simulink model "Linear_acceleration_70"  (R2022a)
settings: Solver=VariableStepAuto  StartTime=0.0  StopTime=inf  RelTol=1e-3
model workspace (MAT data in the model file):
  ratio0 = 2
  ua0 = 4.608
  ua_max = 70
undefined symbols (not defined in the file): CA, f, g, i, i0, If, Iw1, Iw2, kt, m2, r
settings Model: DataDictionary=Vehicle_paramiter.sldd  Creator=cht  LastModifiedBy=cht

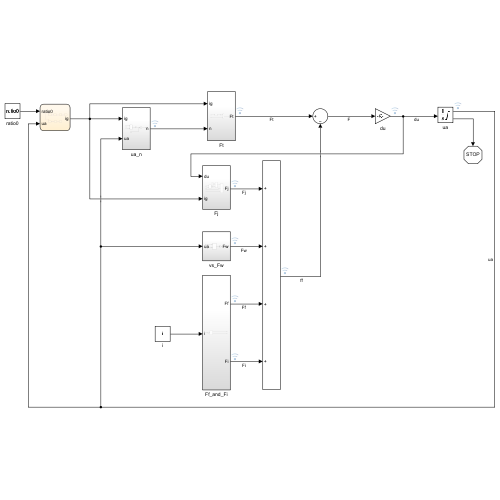
[thumbnail: Simulink's stored preview of the top-level diagram]
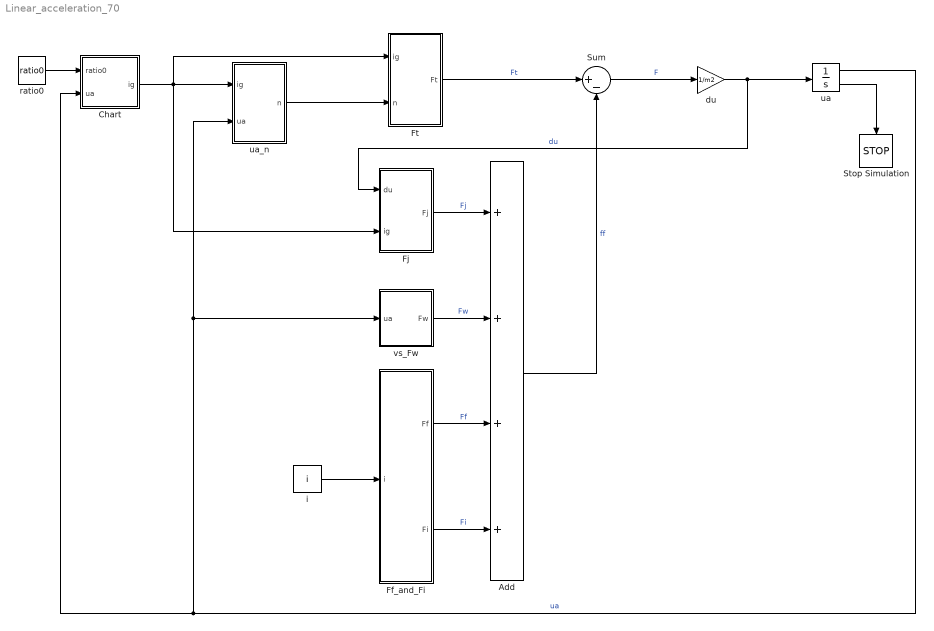
== system Linear_acceleration_70 ==
  Add : Sum  Inputs=++++
  Chart : Stateflow chart  TreatAsAtomicUnit=on
  Ff_and_Fi : Subsystem
  Fj : Subsystem
  Ft : Subsystem
  Stop Simulation : Stop
  Sum : Sum  Inputs=|+-
  du : Gain  Gain=1/m2
  i : Constant  Value=i
  ratio0 : Constant  Value=ratio0
  ua : Integrator  InitialCondition=ua0  LimitOutput=on  UpperSaturationLimit=ua_max  LowerSaturationLimit=0  ShowSaturationPort=on
  ua_n : Subsystem
  vs_Fw : Subsystem
  wires:
  ua_n/1(n) -> Ft/2(n)
  vs_Fw/1(Fw) -> Add/2  "Fw"
  Fj/1(Fj) -> Add/1  "Fj"
  Ff_and_Fi/1(Ff) -> Add/3  "Ff"
  Ff_and_Fi/2(Fi) -> Add/4  "Fi"
  Ft/1(Ft) -> Sum/1  "Ft"
  Add/1 -> Sum/2  "ff"
  Sum/1 -> du/1  "F"
  du/1 -> Fj/1(du), ua/1  "du"
  i/1 -> Ff_and_Fi/1(i)
  ua/1 -> Chart/2(ua), ua_n/2(ua), vs_Fw/1(ua)  "ua"
  ua/2 -> Stop Simulation/1
  Chart/1(ig) -> Fj/2(ig), Ft/1(ig), ua_n/1(ig)
  ratio0/1 -> Chart/1(ratio0)

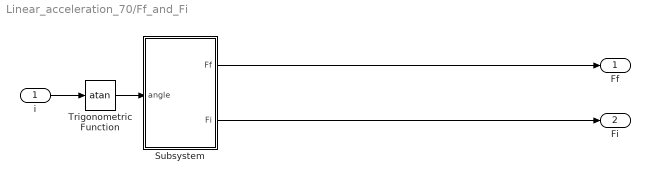
== system Linear_acceleration_70/Ff_and_Fi ==
  i : Inport
  Subsystem : Subsystem
  Trigonometric Function : Trigonometry  Operator=atan
  Ff : Outport
  Fi : Outport  Port=2
  wires:
  i/1 -> Trigonometric Function/1
  Subsystem/1(Ff) -> Ff/1
  Trigonometric Function/1 -> Subsystem/1(angle)
  Subsystem/2(Fi) -> Fi/1

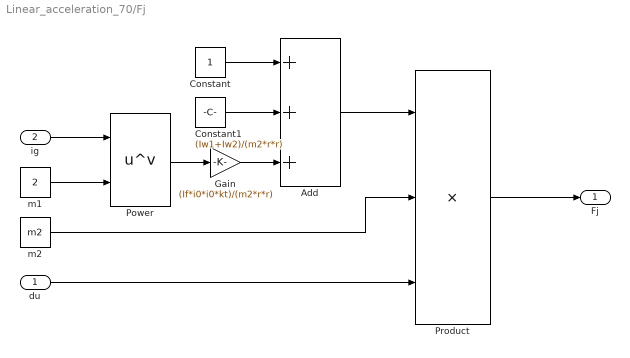
== system Linear_acceleration_70/Fj ==
  du : Inport
  ig : Inport  Port=2
  Add : Sum  Inputs=+++
  Constant : Constant
  Constant1 : Constant  Value=(Iw1+Iw2)/(m2*r*r)
  Gain : Gain  Gain=(If*i0*i0*kt)/(m2*r*r)
  Power : Math  Operator=pow
  Product : Product  Inputs=3
  m1 : Constant  Value=2
  m2 : Constant  Value=m2
  Fj : Outport
  wires:
  Constant1/1 -> Add/2
  Power/1 -> Gain/1
  Gain/1 -> Add/3
  Constant/1 -> Add/1
  du/1 -> Product/3
  ig/1 -> Power/1
  Product/1 -> Fj/1
  Add/1 -> Product/1
  m2/1 -> Product/2
  m1/1 -> Power/2

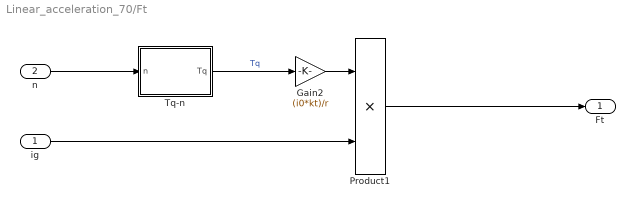
== system Linear_acceleration_70/Ft ==
  ig : Inport
  n : Inport  Port=2
  Gain2 : Gain  Gain=(i0*kt)/r
  Product1 : Product
  Tq-n : MATLAB Function  TreatAsAtomicUnit=on
  Ft : Outport
  wires:
  Product1/1 -> Ft/1
  ig/1 -> Product1/2
  Tq-n/1(Tq) -> Gain2/1  "Tq"
  n/1 -> Tq-n/1(n)
  Gain2/1 -> Product1/1

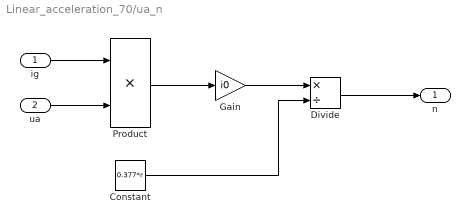
== system Linear_acceleration_70/ua_n ==
  ig : Inport
  ua : Inport  Port=2
  Constant : Constant  Value=0.377*r
  Divide : Product  Inputs=*/
  Gain : Gain  Gain=i0
  Product : Product
  n : Outport
  wires:
  ua/1 -> Product/2
  Product/1 -> Gain/1
  Divide/1 -> n/1
  Constant/1 -> Divide/2
  Gain/1 -> Divide/1
  ig/1 -> Product/1

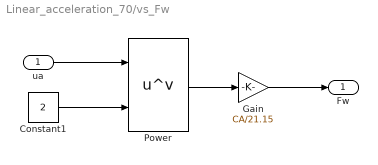
== system Linear_acceleration_70/vs_Fw ==
  ua : Inport
  Constant1 : Constant  Value=2
  Gain : Gain  Gain=CA/21.15
  Power : Math  Operator=pow
  Fw : Outport
  wires:
  Constant1/1 -> Power/2
  Gain/1 -> Fw/1
  ua/1 -> Power/1
  Power/1 -> Gain/1

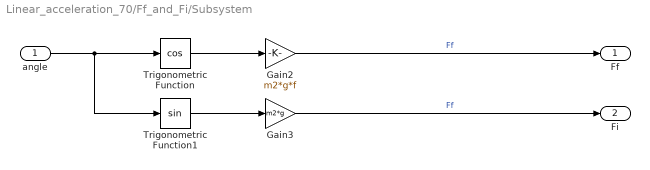
== system Linear_acceleration_70/Ff_and_Fi/Subsystem ==
  angle : Inport
  Gain2 : Gain  Gain=m2*g*f
  Gain3 : Gain  Gain=m2*g
  Trigonometric Function : Trigonometry  Operator=cos
  Trigonometric Function1 : Trigonometry
  Ff : Outport
  Fi : Outport  Port=2
  wires:
  Gain3/1 -> Fi/1  "Ff"
  angle/1 -> Trigonometric Function1/1, Trigonometric Function/1
  Trigonometric Function1/1 -> Gain3/1
  Trigonometric Function/1 -> Gain2/1
  Gain2/1 -> Ff/1  "Ff"

== matlab function Linear_acceleration_70/Ft/Tq-n ==
  data: n input; Tq output
function Tq = fcn(n)
%#codegen

Tq = -19.313+295.27*(n/1000)-165.44*(n/1000)^2+40.874*(n/1000)^3-3.8445*(n/1000)^4;

== stateflow chart Linear_acceleration_70/Chart ==
  state ratio1
    en:
    ig=6.09
  state ratio2
    en:
    ig=3.09
  state ratio3
    en:
    ig=1.71
  state ratio4
    en:
    ig=1
  state ratio2_2
    en:
    ig=3.09
  state ratio2_3
    en:
    ig=1.71
  state ratio2_4
    en:
    ig=1
  (default) -> (junction 4)
  (junction 4) -> (junction 8) [order 1]
  (junction 4) -> (junction 5) [order 2]
  (junction 8) -> ratio1 : [ratio0==1]
  ratio1 -> ratio2 : [ua>15]
  ratio2 -> ratio3 [order 1] : [ua>30]
  ratio3 -> ratio4 [order 1] : [ua>55]
  ratio2 -> ratio1 [order 2] : [ua<14]
  ratio4 -> ratio3 : [ua<50]
  ratio3 -> ratio2 [order 2] : [ua<25]
  (junction 5) -> (junction 10)
  (junction 10) -> ratio2_2
  ratio2_2 -> ratio2_3 : [ua>30]
  ratio2_3 -> ratio2_4 [order 1] : [ua>55]
  ratio2_4 -> ratio2_3 : [ua<50]
  ratio2_3 -> ratio2_2 [order 2] : [ua<25]
  data: ratio0 input; ig output; ua input
